simulink model "model_best_result"  (R2018b)
settings: Solver=VariableStepAuto  StartTime=0.0  StopTime=4000  FixedStep=1e-4  RelTol=1e-3
undefined symbols (not defined in the file): a, b, d, sigbuilder_block
libraries: powerlib x6
settings Model: Creator=Mihai  LastModifiedBy=Mihai

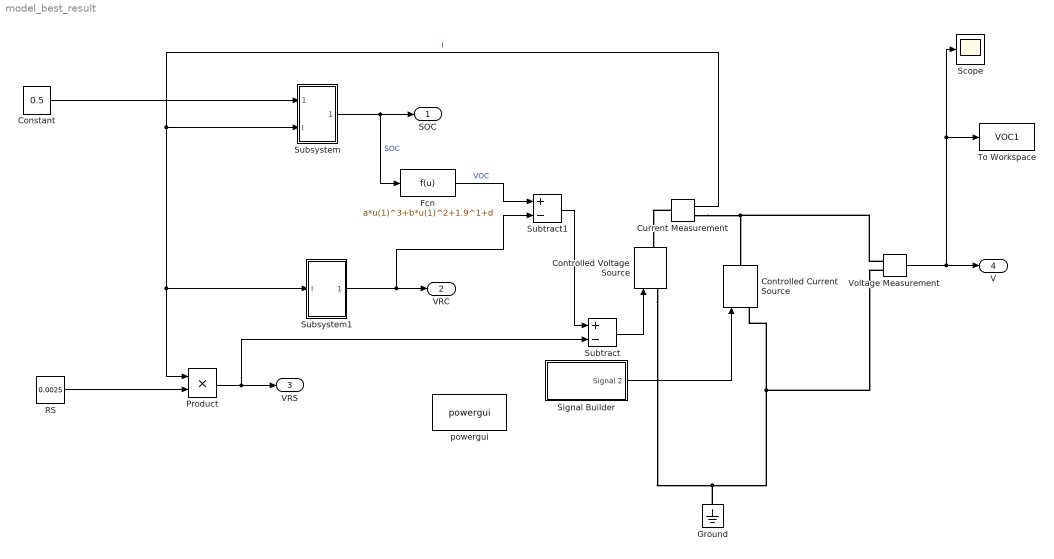
== system model_best_result ==
  Constant : Constant  Value=0.5
  Controlled Current Source : powerlib/Electrical Sources/Controlled Current Source  Initialize=on  Source_Type=DC  Amplitude=0  Phase=0  Frequency=0  Measurements=None
  Controlled Voltage Source : powerlib/Electrical Sources/Controlled Voltage Source  Initialize=on  Source_Type=DC  Amplitude=0  Phase=0  Frequency=0  Measurements=None
  Current Measurement : powerlib/Measurements/Current Measurement  PhasorSimulation=off  OutputType=Complex  PSBequivalent=0
  Fcn : Fcn  Expr=a*u(1)^3+b*u(1)^2+1.9^1+d
  Ground : powerlib/Elements/Ground  LConnTagsString=a
  Product : Product
  RS : Constant  Value=0.0025
  Scope : Scope
  Signal Builder : Subsystem  Tag=STV Subsys  LoadFcn=sigbuilder_block('load',[576.6 30.6 574.8 555.6 ]);  StartFcn=sigbuilder_block('start');  StopFcn=sigbuilder_block('stop');  ClipboardFcn=sigbuilder_block('clipboard');  mask(Sigbuilder block){tuvar=[0:10]}
      mask help: Simulink:masks:SigbuilderBlock_MD
      mask init:
      | if ~strcmp(get_param(bdroot(gcbh),'SimulationStatus'),'stopped') tuvar = sigbuilder_block('maskInit'); end
      settings: CopyFcn=sigbuilder_block('copy');  DeleteFcn=sigbuilder_block('delete');  ModelCloseFcn=sigbuilder_block('modelClose');  PreSaveFcn=sigbuilder_block('preSave');  PauseFcn=sigbuilder_block('pause');  ContinueFcn=sigbuilder_block('continue');  NameChangeFcn=sigbuilder_block('namechange');  OpenFcn=sigbuilder_block('open',[5.4 31.8 1141.2 483.6 ]);  CloseFcn=sigbuilder_block('close');
      mask Display: plot(0, 0, 100, 100,[2, 2, 32, 32, 2], [68, 8, 8, 68, 68],[32, 2], [38, 38], [32, 19, 2],[53, 60, 44], [32, 17, 17, 2],[16, 16, 31, 31]);txt = getActiveGroup(gcbh);text(2, 100, txt,'verticalAlignment', 'top');
  Subsystem : Subsystem
  Subsystem1 : Subsystem
  Subtract : Sum  Inputs=+-
  Subtract1 : Sum  Inputs=+-
  To Workspace : ToWorkspace  VariableName=VOC1  SaveFormat=Timeseries  SampleTime=-1
  Voltage Measurement : powerlib/Measurements/Voltage Measurement  PhasorSimulation=off  OutputType=Complex  PSBequivalent=0
  powergui : powerlib/powergui  Priority=1  SimulationMode=Continuous  SampleTime=5e-3  frequency=60  Iterations=50  frequencyindice=0  Pbase=100e6  ErrMax=1e-4  UnitsV=kV  UnitsW=MW  buscounter=0  FunctionMessages=off  echomessages=off  EnableUseOfTLC=off  CurrentSourceSwitches=off  DisableSnubberDevices=off  DisableRonSwitches=off  DisableVfSwitches=off  DisplayEquations=off  SolverType=Tustin/Backward Euler (TBE)  Interpol=off  ExternalGateDelay=off  methode=off  Ts=100  x0status=blocks  SPID=off  SwTol=0  HookPort=off  RestoreLinks=warning  ResistiveCurrentMeasurement=off  Frange=[0:2:500]  Ylog=off  Xlog=on  ShowGrid=off  save=off  variable=ZData  structure=0  ZoomFFT=off  StartTime=0.0  cycles=1  DisplayStyle=1  fundamental=60  FreqAxis=off  MaxFrequency=1000  frequencyindicesteady=1  RmsSteady=1  display=off
  SOC : Outport
  VRC : Outport  Port=2
  VRS : Outport  Port=3
  V : Outport  Port=4
  wires:
  Constant/1 -> Subsystem/1(SOC0)
  Subsystem/1(SOC) -> SOC/1, Fcn/1  "SOC"
  Current Measurement/1 -> Product/1, Subsystem1/1(I), Subsystem/2(I)  "I"
  Subsystem1/1(VRC) -> Subtract1/2, VRC/1
  RS/1 -> Product/2
  Product/1 -> Subtract/2, VRS/1
  Fcn/1 -> Subtract1/1  "VOC"
  Subtract1/1 -> Subtract/1
  Subtract/1 -> Controlled Voltage Source/1
  Voltage Measurement/1 -> V/1, To Workspace/1, Scope/1
  Signal Builder/1(Signal 2) -> Controlled Current Source/1
  connections:
  Current Measurement/LConn1 -- Controlled Voltage Source/RConn1
  Current Measurement/RConn1 -- Controlled Current Source/RConn1 -- Voltage Measurement/LConn1
  Controlled Voltage Source/LConn1 -- Ground/LConn1 -- Controlled Current Source/LConn1 -- Voltage Measurement/LConn2

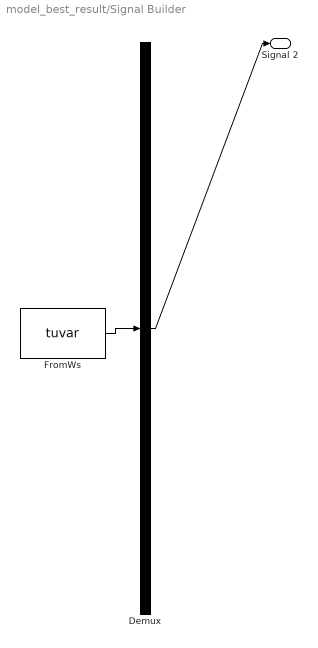
== system model_best_result/Signal Builder ==
  Demux : Demux  Tag=STV Demux  Outputs=1
  FromWs : FromWorkspace  Tag=STV FromWs  VariableName=tuvar  SampleTime=0
      SigBuilderData=|
      | common.afterFinalStr = 'Extrapolate'
      | common.sampleTime = 0
      | dataSet.timeRange = [0 2000]
      | dataSet.name = 'Group 1'
      | sbobj.Groups.Name = 'Group 1'
      | sbobj.Groups.Signals.Name = 'Signal 2'
      | sbobj.Groups.Signals.XData = [0 405 405 800 800 2000]
      | sbobj.Groups.Signals.YData = [0 0 -10 -10 0 0]
      | sbobj.Groups.TimeRange = [0 2000]
  Signal 2 : Outport  Tag=STV Outport
  wires:
  FromWs/1 -> Demux/1
  Demux/1 -> Signal 2/1

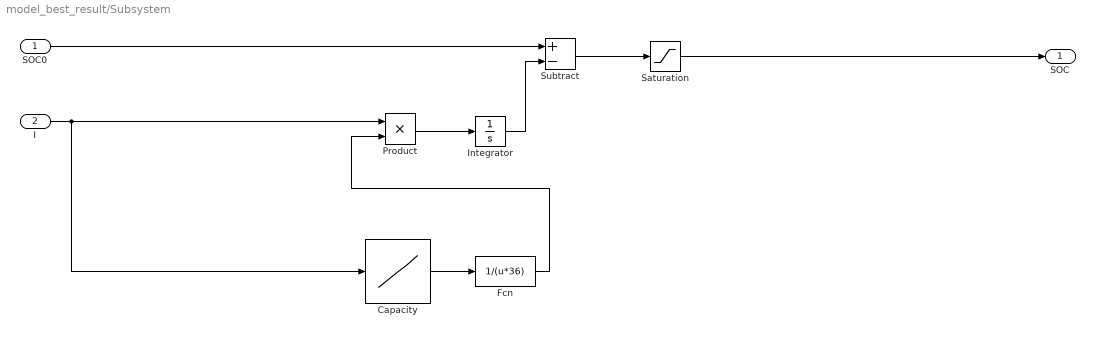
== system model_best_result/Subsystem ==
  SOC0 : Inport
  I : Inport  Port=2
  Capacity : Lookup_n-D  NumberOfTableDimensions=1  BreakpointsForDimension1=[0 10]  Table=[19.3 0]  InternalRulePriority=Speed  RndMeth=Simplest  InputSameDT=on
  Fcn : Fcn  Expr=1/(u*36)
  Integrator : Integrator
  Product : Product
  Saturation : Saturate  UpperLimit=1  LowerLimit=0
  Subtract : Sum  Inputs=+-
  SOC : Outport
  wires:
  Product/1 -> Integrator/1
  Integrator/1 -> Subtract/2
  I/1 -> Capacity/1, Product/1
  SOC0/1 -> Subtract/1
  Fcn/1 -> Product/2
  Capacity/1 -> Fcn/1
  Subtract/1 -> Saturation/1
  Saturation/1 -> SOC/1

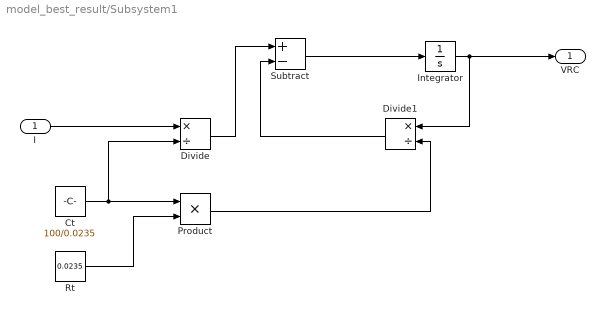
== system model_best_result/Subsystem1 ==
  I : Inport
  Ct : Constant  Value=100/0.0235
  Divide : Product  Inputs=*/
  Divide1 : Product  Inputs=*/
  Integrator : Integrator
  Product : Product
  Rt : Constant  Value=0.0235
  Subtract : Sum  Inputs=+-
  VRC : Outport
  wires:
  Ct/1 -> Divide/2, Product/1
  Integrator/1 -> VRC/1, Divide1/1
  Rt/1 -> Product/2
  I/1 -> Divide/1
  Subtract/1 -> Integrator/1
  Product/1 -> Divide1/2
  Divide1/1 -> Subtract/2
  Divide/1 -> Subtract/1
